simulink model "pi_aliasIface"  (R2018b)
settings: Solver=FixedStepDiscrete  StartTime=0.0  StopTime=10.0  RelTol=1e-3
undefined symbols (not defined in the file): arr, nCount
settings Model: Creator=matlab  LastModifiedBy=matlab
settings DataIOCC: SaveOutput=off  SignalLogging=off  SaveTime=off
settings OptimizationCC: DefaultParameterBehavior=Inlined  EnhancedBackFolding=on  PassReuseOutputArgsAs=Individual arguments  OptimizeBlockOrder=speed  DifferentSizesBufferReuse=on  OptimizationCustomize=off
settings DebuggingCC: ParameterTunabilityLossMsg=error
settings SFSimCC: MATLABDynamicMemAlloc=off
settings RTWCC: SystemTargetFile=ert.tlc  TemplateMakefile=ert_default_tmf  PostCodeGenCommand=packNGo(buildInfo);  GenerateReport=on  IncludeHyperlinkInReport=on  LaunchReport=on  GenerateTraceInfo=on  GenerateTraceReport=on  GenerateTraceReportSl=on  GenerateTraceReportSf=on  GenerateTraceReportEml=on
settings CodeAppCC: ForceParamTrailComments=on  IgnoreCustomStorageClasses=off  OperatorAnnotations=on  SimulinkDataObjDesc=on  SFDataObjDesc=on  InsertBlockDesc=on
settings ERTTargetCC: TargetLangStandard=C99 (ISO)  GenerateSampleERTMain=on  InlinedParameterPlacement=NonHierarchical  ERTCustomFileTemplate=example_file_process.tlc

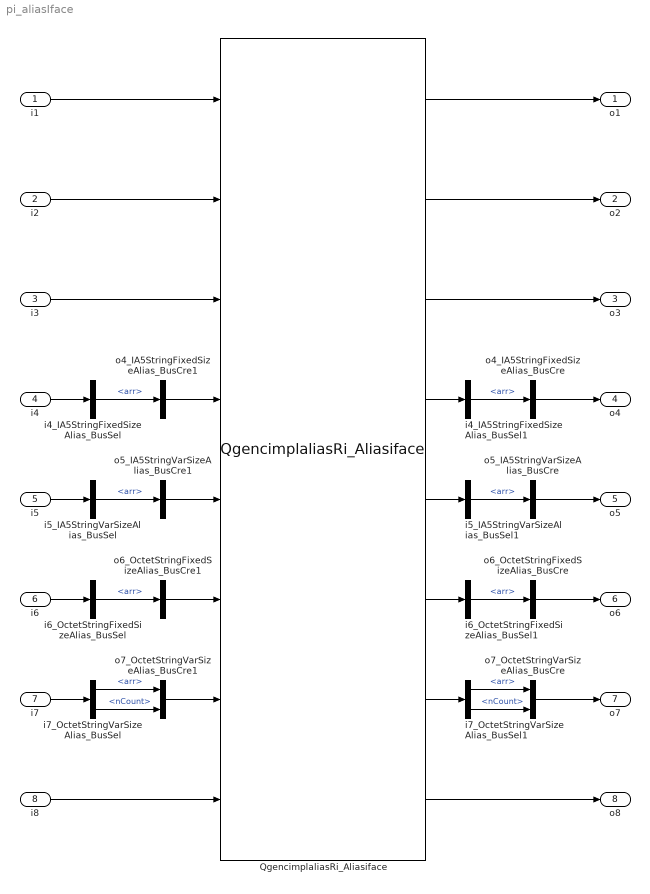
== system pi_aliasIface ==
  i1 : Inport  OutDataTypeStr=BoolAlias  BusOutputAsStruct=on
  i2 : Inport  Port=2  OutDataTypeStr=IntegerAlias  BusOutputAsStruct=on
  i3 : Inport  Port=3  OutDataTypeStr=RealAlias  BusOutputAsStruct=on
  i4 : Inport  Port=4  OutDataTypeStr=Bus: IA5StringFixedSizeAlias  BusOutputAsStruct=on
  i5 : Inport  Port=5  OutDataTypeStr=Bus: IA5StringVarSizeAlias  BusOutputAsStruct=on
  i6 : Inport  Port=6  OutDataTypeStr=Bus: OctetStringFixedSizeAlias  BusOutputAsStruct=on
  i7 : Inport  Port=7  OutDataTypeStr=Bus: OctetStringVarSizeAlias  BusOutputAsStruct=on
  i8 : Inport  Port=8  OutDataTypeStr=Enum: EnumAlias  BusOutputAsStruct=on
  QgencimplaliasRi_Aliasiface : S-Function  FunctionName=QgencimplaliasRi_Aliasiface  SFunctionDeploymentMode=off  EnableBusSupport=off  mask(Legacy Function){SFunctionSpec=void qgencimplalias_RI_ri_aliasIface(BoolAlias u1[1], IntegerAlias u2[1], RealAlias u3[1], IA5StringFixedSizeAlias u4[1], IA5StringVarSizeAlias u5[1], OctetStringFixedSizeAlias u6[1], OctetStringVarSizeAlias u7[1], EnumAlias u8[1], BoolAlias y1[1], IntegerAlias y2[1], RealAlias y3[1], IA5StringFixedSizeAlias y4[1], IA5StringVarSizeAlias y5[1], OctetStringFixedSizeAlias y6[1], OctetStringVarSizeAlias y7[1], EnumAlias y8[1]), ShowSpec=off}
      mask prompts: ShowSpec "Display function specification"
      mask help:
      | This block allows you to call the legacy functions specified by the following Legacy Code Tool definition:
      | def.SFunctionName = 'QgencimplaliasRi_Aliasiface';
      | def.OutputFcnSpec = 'void qgencimplalias_RI_ri_aliasIface(BoolAlias u1[1], IntegerAlias u2[1], RealAlias u3[1], IA5StringFixedSizeAlias u4[1], IA5StringVarSizeAlias u5[1], OctetStringFixedSizeAlias u6[1], OctetStringVarSizeAlias u7[1], EnumAlias u8[1], BoolAlias y1[1], IntegerAlias y2[1], RealAlias y3[1], IA5StringFixedSizeAlias y4[1], IA5StringVarSizeAlias y5[1], OctetStringFixedSizeAlias y6[1], OctetStringVarSizeAlias y7[1], EnumAlias y8[1])';
      | def.HeaderFiles = {'qgencimplalias_invoke_ri.h'};
      | def.SourceFiles = {'qgencimplalias_invoke_ri.c'};
      | def.IncPaths = {'..\..\..\dataview\C'};
      mask Help: <p>This block was generated automatically by the Legacy Code Tool. For detailed help on this tool, call<a href="matlab:legacy_code('help')"> legacy_code('help')</a>.</p>
      mask Callback ShowSpec:
      | if strcmp(get_param(gcbh, 'ShowSpec'), 'on')
      |   set_param(gcbh, 'MaskDisplay', sprintf('fprintf(''%s'');', get_param(gcbh, 'SFunctionSpec')));
      | else
      |   set_param(gcbh, 'MaskDisplay', sprintf('fprintf(''%s'');', get_param(gcbh, 'FunctionName')));
      | end
      mask Display: fprintf('QgencimplaliasRi_Aliasiface');
  i4_IA5StringFixedSizeAlias_BusSel : BusSelector  OutputSignals=arr
  i4_IA5StringFixedSizeAlias_BusSel1 : BusSelector  OutputSignals=arr
  i5_IA5StringVarSizeAlias_BusSel : BusSelector  OutputSignals=arr
  i5_IA5StringVarSizeAlias_BusSel1 : BusSelector  OutputSignals=arr
  i6_OctetStringFixedSizeAlias_BusSel : BusSelector  OutputSignals=arr
  i6_OctetStringFixedSizeAlias_BusSel1 : BusSelector  OutputSignals=arr
  i7_OctetStringVarSizeAlias_BusSel : BusSelector  OutputSignals=arr,nCount
  i7_OctetStringVarSizeAlias_BusSel1 : BusSelector  OutputSignals=arr,nCount
  o4_IA5StringFixedSizeAlias_BusCre : BusCreator  Inputs=1  OutDataTypeStr=Bus: IA5StringFixedSizeAlias  NonVirtualBus=on
  o4_IA5StringFixedSizeAlias_BusCre1 : BusCreator  Inputs=1  OutDataTypeStr=Bus: IA5StringFixedSizeAlias  NonVirtualBus=on
  o5_IA5StringVarSizeAlias_BusCre : BusCreator  Inputs=1  OutDataTypeStr=Bus: IA5StringVarSizeAlias  NonVirtualBus=on
  o5_IA5StringVarSizeAlias_BusCre1 : BusCreator  Inputs=1  OutDataTypeStr=Bus: IA5StringVarSizeAlias  NonVirtualBus=on
  o6_OctetStringFixedSizeAlias_BusCre : BusCreator  Inputs=1  OutDataTypeStr=Bus: OctetStringFixedSizeAlias  NonVirtualBus=on
  o6_OctetStringFixedSizeAlias_BusCre1 : BusCreator  Inputs=1  OutDataTypeStr=Bus: OctetStringFixedSizeAlias  NonVirtualBus=on
  o7_OctetStringVarSizeAlias_BusCre : BusCreator  Inputs=arr,nCount  OutDataTypeStr=Bus: OctetStringVarSizeAlias  NonVirtualBus=on
  o7_OctetStringVarSizeAlias_BusCre1 : BusCreator  Inputs=arr,nCount  OutDataTypeStr=Bus: OctetStringVarSizeAlias  NonVirtualBus=on
  o1 : Outport  OutDataTypeStr=BoolAlias
  o2 : Outport  Port=2  OutDataTypeStr=IntegerAlias
  o3 : Outport  Port=3  OutDataTypeStr=RealAlias
  o4 : Outport  Port=4  OutDataTypeStr=Bus: IA5StringFixedSizeAlias  BusOutputAsStruct=on
  o5 : Outport  Port=5  OutDataTypeStr=Bus: IA5StringVarSizeAlias  BusOutputAsStruct=on
  o6 : Outport  Port=6  OutDataTypeStr=Bus: OctetStringFixedSizeAlias  BusOutputAsStruct=on
  o7 : Outport  Port=7  OutDataTypeStr=Bus: OctetStringVarSizeAlias  BusOutputAsStruct=on
  o8 : Outport  Port=8  OutDataTypeStr=Enum: EnumAlias
  wires:
  i4/1 -> i4_IA5StringFixedSizeAlias_BusSel/1
  i5/1 -> i5_IA5StringVarSizeAlias_BusSel/1
  i6/1 -> i6_OctetStringFixedSizeAlias_BusSel/1
  i7/1 -> i7_OctetStringVarSizeAlias_BusSel/1
  o4_IA5StringFixedSizeAlias_BusCre/1 -> o4/1
  o5_IA5StringVarSizeAlias_BusCre/1 -> o5/1
  o6_OctetStringFixedSizeAlias_BusCre/1 -> o6/1
  o7_OctetStringVarSizeAlias_BusCre/1 -> o7/1
  o6_OctetStringFixedSizeAlias_BusCre1/1 -> QgencimplaliasRi_Aliasiface/6
  o5_IA5StringVarSizeAlias_BusCre1/1 -> QgencimplaliasRi_Aliasiface/5
  o4_IA5StringFixedSizeAlias_BusCre1/1 -> QgencimplaliasRi_Aliasiface/4
  o7_OctetStringVarSizeAlias_BusCre1/1 -> QgencimplaliasRi_Aliasiface/7
  i4_IA5StringFixedSizeAlias_BusSel/1 -> o4_IA5StringFixedSizeAlias_BusCre1/1  "<arr>"
  i5_IA5StringVarSizeAlias_BusSel/1 -> o5_IA5StringVarSizeAlias_BusCre1/1  "<arr>"
  i6_OctetStringFixedSizeAlias_BusSel/1 -> o6_OctetStringFixedSizeAlias_BusCre1/1  "<arr>"
  i7_OctetStringVarSizeAlias_BusSel/1 -> o7_OctetStringVarSizeAlias_BusCre1/1  "<arr>"
  i7_OctetStringVarSizeAlias_BusSel/2 -> o7_OctetStringVarSizeAlias_BusCre1/2  "<nCount>"
  i6_OctetStringFixedSizeAlias_BusSel1/1 -> o6_OctetStringFixedSizeAlias_BusCre/1  "<arr>"
  i7_OctetStringVarSizeAlias_BusSel1/1 -> o7_OctetStringVarSizeAlias_BusCre/1  "<arr>"
  i4_IA5StringFixedSizeAlias_BusSel1/1 -> o4_IA5StringFixedSizeAlias_BusCre/1  "<arr>"
  QgencimplaliasRi_Aliasiface/4 -> i4_IA5StringFixedSizeAlias_BusSel1/1
  QgencimplaliasRi_Aliasiface/5 -> i5_IA5StringVarSizeAlias_BusSel1/1
  i5_IA5StringVarSizeAlias_BusSel1/1 -> o5_IA5StringVarSizeAlias_BusCre/1  "<arr>"
  i7_OctetStringVarSizeAlias_BusSel1/2 -> o7_OctetStringVarSizeAlias_BusCre/2  "<nCount>"
  QgencimplaliasRi_Aliasiface/7 -> i7_OctetStringVarSizeAlias_BusSel1/1
  QgencimplaliasRi_Aliasiface/6 -> i6_OctetStringFixedSizeAlias_BusSel1/1
  i1/1 -> QgencimplaliasRi_Aliasiface/1
  QgencimplaliasRi_Aliasiface/8 -> o8/1
  i2/1 -> QgencimplaliasRi_Aliasiface/2
  i3/1 -> QgencimplaliasRi_Aliasiface/3
  QgencimplaliasRi_Aliasiface/1 -> o1/1
  QgencimplaliasRi_Aliasiface/2 -> o2/1
  QgencimplaliasRi_Aliasiface/3 -> o3/1
  i8/1 -> QgencimplaliasRi_Aliasiface/8
